simulink model "Vectored_Thruster"  (R2021b)
settings: Solver=VariableStepAuto  StartTime=0.0  StopTime=50  FixedStep=0.0001  RelTol=1e-3
undefined symbols (not defined in the file): X, Y, Z
libraries: sm_lib x59, nesl_utility x10, slpidlib x4, checkpacklib x1
(part 3 of 3)

== matlab function Vectored_Thruster/MATLAB Function ==
  data: e1 input; y output; e2 input; e3 input
function y = fcn(e1,e2,e3)
y=0;

if -0.005<e1 && e1<0.005 && -0.005<e2 && e2<0.005 && -0.005<e3 && e3<0.005
    y=1;
end

end

== matlab function Vectored_Thruster/Inverse Kinematics ==
  data: R input; r input; cz input; l1 output; beta input; theta input; l2 output; l3 output
function [l1,l2,l3] = fcn(R,r,cz,beta,theta)
alpha=atan((sind(beta)*sind(theta))/(cosd(beta)+cosd(theta)));
a=cosd(alpha)*cosd(beta);
b=cosd(alpha)*sind(beta)*sind(theta)-sind(alpha)*cosd(theta);
c=cosd(alpha)*sind(beta)*cosd(theta)+sind(alpha)*sind(theta);
d=sind(alpha)*cosd(beta);
e=sind(alpha)*sind(beta)*sind(theta)+cosd(alpha)*cosd(theta);
f=sind(alpha)*sind(beta)*cosd(theta)-cosd(alpha)*sind(theta);
g=-sind(beta);
h=cosd(beta)*sind(theta);
i=cosd(beta)*cosd(theta);
Rot=[a,b,c;d,e,f;g,h,i];
B1c=[r;0;0];
B2c=[-r/2;(-r*1.732)/2;0];
B3c=[-r/2;(r*1.732)/2;0];

A1=[R;0;0];
A2=[-R/2;(-R*1.732)/2;0];
A3=[-R/2;(R*1.732)/2;0];

cx=((-r/2))*(cosd(alpha)*cosd(theta)-(sind(alpha)*sind(beta)*sind(theta))-(cosd(beta)*cosd(theta)));
cy=-r*sind(alpha)*cosd(beta) ;
c=[cx;cy;cz];

B1=Rot*B1c + c;
B2=Rot*B2c + c;
B3=Rot*B3c + c;

l1=norm(B1-A1)-0.131;
l2=norm(B2-A2)-0.131;
l3=norm(B3-A3)-0.131;
end

== matlab function Vectored_Thruster/Thrust & LinearSpeed Calculator/Linearspeed Calc ==
  data: vel input; linearspeed output; efficiency output
function [linearspeed,efficiency] = fcn(vel)
pitch_angle= 45;
prop_d=0.15;
pitch= tand(pitch_angle)*prop_d*pi;
rpm=vel*30/pi;
if(rpm<10)
    efficiency=0.1;
elseif(rpm<20)
    efficiency=0.2;
elseif(rpm<30)
    efficiency=0.3; 
elseif(rpm<40)
    efficiency=0.4;
elseif(rpm<50)
    efficiency=0.5;
elseif(rpm<100)
    efficiency=0.6;
else
    efficiency=0.7;
end
linearspeed=pitch*efficiency*rpm/60;
end

== matlab function Vectored_Thruster/Thrust & LinearSpeed Calculator/MATLAB Function ==
  data: vel input; thrust output; torque input; efficiency input; linearspeed input
function thrust = fcn(vel, torque,efficiency,linearspeed)
thrust=vel*torque*efficiency/0.1+linearspeed;
end
